simulink model "Lorenz_SysID_example"  (R2019a)
settings: Solver=ode23t  StartTime=0.0  StopTime=100  RelTol=1e-3
settings Model: Creator=jxs210080  LastModifiedBy=jxs210080
settings DebuggingCC: UnconnectedInputMsg=none  UnconnectedOutputMsg=none  UnconnectedLineMsg=none
settings ModelReferenceCC: EnableRefExpFcnMdlSchedulingChecks=off
settings RTWCC: Description=Generic Real-Time Target

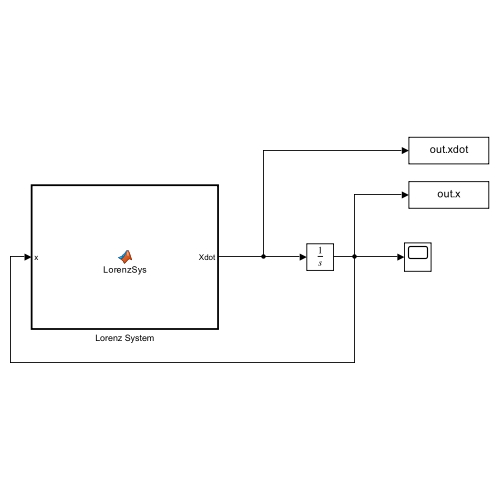
[thumbnail: Simulink's stored preview of the top-level diagram]
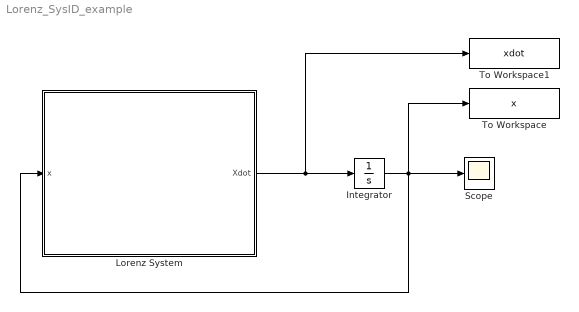
== system Lorenz_SysID_example ==
  Integrator : Integrator  InitialCondition=[0;1;20]
  Lorenz System : MATLAB Function  TreatAsAtomicUnit=on
  Scope : Scope
  To Workspace : ToWorkspace  VariableName=x  SaveFormat=Timeseries  SampleTime=-1
  To Workspace1 : ToWorkspace  VariableName=xdot  SaveFormat=Timeseries  SampleTime=-1
  wires:
  Lorenz System/1(Xdot) -> To Workspace1/1, Integrator/1
  Integrator/1 -> To Workspace/1, Scope/1, Lorenz System/1(x)

== matlab function Lorenz_SysID_example/Lorenz System ==
  data: x input; Xdot output
function Xdot = LorenzSys(x)

% System Parameters
sigma = 10;
rho = 28;
beta = 8/3;

% System Dynamics

x1_dot = sigma*(x(2) - x(1));
x2_dot = x(1)*(rho - x(3)) - x(2);
x3_dot = (x(1)*x(2)) - (beta*x(3));

Xdot = [x1_dot; x2_dot; x3_dot];

end
